simulink model "test_model"  (R2020b)
settings: Solver=FixedStepAuto  StartTime=0.0  StopTime=inf  FixedStep=0.001  RelTol=1e-3
libraries: DSX_Lib x15
settings Model: PacingRate=0.450000  Creator=16047  LastModifiedBy=16047
settings DebuggingCC: InheritedTsInSrcMsg=none

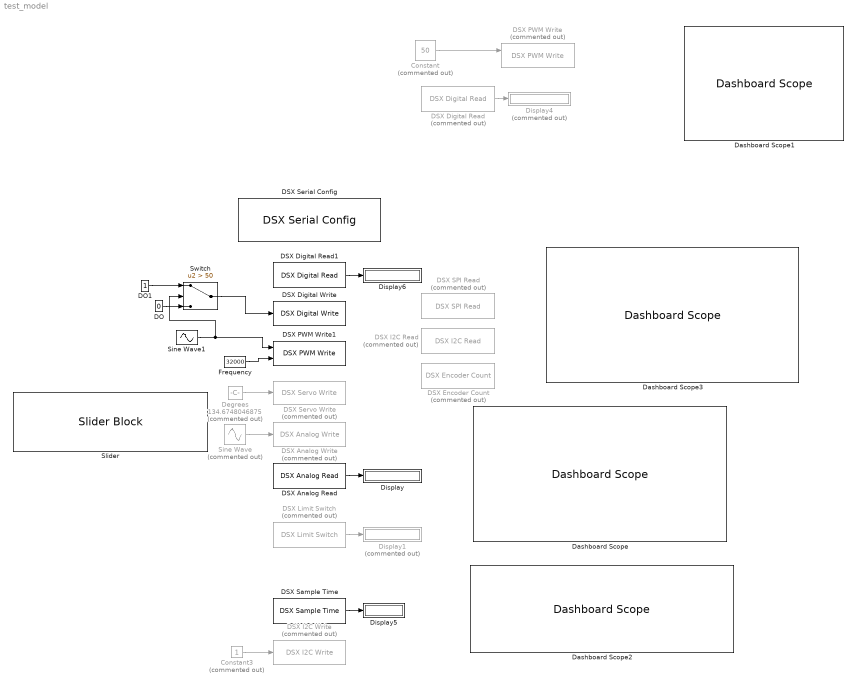
== system test_model ==
  Constant : Constant  Commented=on  Value=50
  Constant3 : Constant  Commented=on
  DO : Constant  Value=0
  DO1 : Constant
  DSX Analog Read : DSX_Lib/Read Blocks/DSX Analog Read  aread_pin=13
      settings: SourceProductName=DSX Library
  DSX Analog Write : DSX_Lib/Write Blocks/DSX Analog Write  Commented=on  analog_pin=17
      settings: SourceProductName=DSX Library
  DSX Digital Read : DSX_Lib/Read Blocks/DSX Digital Read  Commented=on  read_pin=1
      settings: SourceProductName=DSX Library
  DSX Digital Read1 : DSX_Lib/Read Blocks/DSX Digital Read  read_pin=2
      settings: SourceProductName=DSX Library
  DSX Digital Write : DSX_Lib/Write Blocks/DSX Digital Write  gpio_pin=9
      settings: SourceProductName=DSX Library
  DSX Encoder Count : DSX_Lib/Read Blocks/DSX Encoder Count  Commented=on  eread_CPR=999
      settings: SourceProductName=DSX Library
  DSX I2C Read : DSX_Lib/Read Blocks/DSX I2C Read  Commented=on  i2c_slave=0
      settings: SourceProductName=DSX Library
  DSX I2C Write : DSX_Lib/Write Blocks/DSX I2C Write  Commented=on  i2c_id=0  i2c_spec=Position  i2c_comp=on
      settings: SourceProductName=DSX Library
  DSX Limit Switch : DSX_Lib/Read Blocks/DSX Limit Switch  Commented=on  read_pin=7  emerg_stop=on
      settings: SourceProductName=DSX Library
  DSX PWM Write : DSX_Lib/Write Blocks/DSX PWM Write  Commented=on  pwm_pin=11  pwm_freq=4000
      settings: SourceProductName=DSX Library
  DSX PWM Write1 : DSX_Lib/Write Blocks/DSX PWM Write  pwm_pin=11  pwm_freq=4000
      settings: SourceProductName=DSX Library
  DSX SPI Read : DSX_Lib/Read Blocks/DSX SPI Read  Commented=on
      settings: SourceProductName=DSX Library
  DSX Sample Time : DSX_Lib/Read Blocks/DSX Sample Time
      settings: SourceProductName=DSX Library
  DSX Serial Config : DSX_Lib/DSX Serial Config  BaudRate=230400
      settings: SourceProductName=DSX Library
  DSX Servo Write : DSX_Lib/Write Blocks/DSX Servo Write  Commented=on  servo_pin=11  servo_min=0  servo_max=180
      settings: SourceProductName=DSX Library
  Dashboard Scope : DashboardScope  Ymin=0  Ymax=8500
  Dashboard Scope1 : DashboardScope
  Dashboard Scope2 : DashboardScope  Ymin=0  Ymax=1
  Dashboard Scope3 : DashboardScope  TimeSpan=1  Ymin=0  Ymax=100
  Degrees : Constant  Commented=on  Value=134.6748046875
  Display : Display
  Display1 : Display  Commented=on
  Display4 : Display  Commented=on
  Display5 : Display
  Display6 : Display
  Frequency : Constant  Value=32000  VectorParams1D=off
  Sine Wave : Sin  Commented=on  Amplitude=1024  Bias=1024  Frequency=0.05  SampleTime=0
  Sine Wave1 : Sin  Amplitude=50  Bias=50  Frequency=10  SampleTime=0
  Slider : SliderBlock  ScaleMax=180
  Switch : Switch  Criteria=u2 > Threshold  Threshold=50
  wires:
  Constant/1 -> DSX PWM Write/1
  DSX Analog Read/1 -> Display/1
  Sine Wave/1 -> DSX Analog Write/1
  DSX Limit Switch/1 -> Display1/1
  Sine Wave1/1 -> Switch/2, DSX PWM Write1/1
  Frequency/1 -> DSX PWM Write1/2
  Constant3/1 -> DSX I2C Write/1
  DSX Digital Read/1 -> Display4/1
  DSX Sample Time/1 -> Display5/1
  Degrees/1 -> DSX Servo Write/1
  DSX Digital Read1/1 -> Display6/1
  DO/1 -> Switch/3
  Switch/1 -> DSX Digital Write/1
  DO1/1 -> Switch/1
